simulink model "simulink_model"  (R2024a)
settings: Solver=VariableStepAuto  StartTime=0.0  StopTime=1  RelTol=1e-3
values from neighbouring files (symbols this model uses):
  control = set_control_gain(Kt_history(pid_count), input, control)    [Kd_tuner.m]    (also in Kd_tuner_newton.m = set_control_gain(Kt_history(pid_count)+delta_x, input, contr; target_tuner.m = set_control_gain(Kp_init, input, control))
undefined symbols (not defined in the file or in its folder): DiscIntNeverNeededParam, input, model
libraries: simulink x5, slpidlib x2
settings Model: PacingRate=0.010000  Creator=dionl  LastModifiedBy=dionl

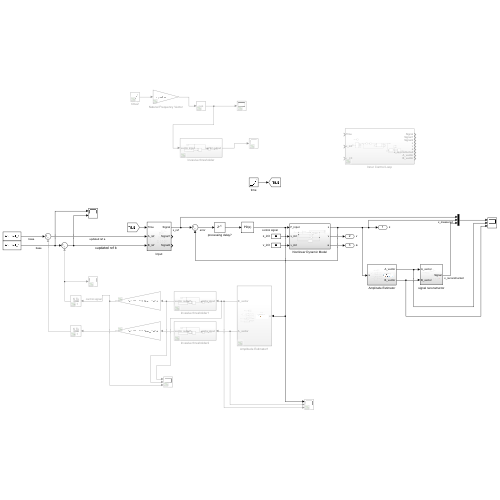
[thumbnail: Simulink's stored preview of the top-level diagram]
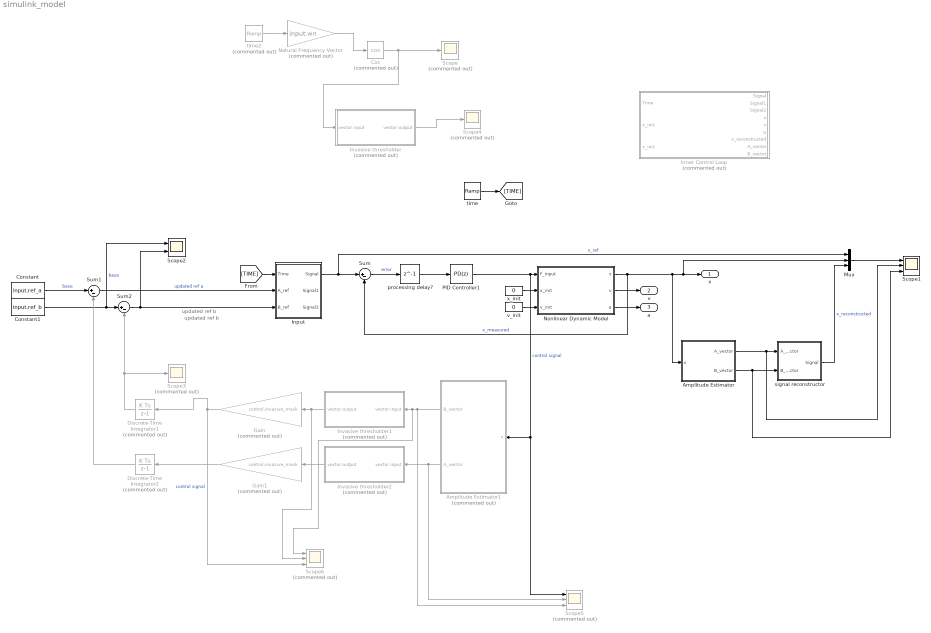
== system simulink_model ==
  note: updated ref b
  note: updated ref b
  Amplitude Estimator : Subsystem
  Amplitude Estimator1 : Subsystem  Commented=on
  Constant : Constant  Value=input.ref_a
  Constant1 : Constant  Value=input.ref_b
  Cos : Trigonometry  Commented=on  Operator=cos
  Discrete-Time Integrator1 : DiscreteIntegrator  Commented=on  SampleTime=input.T0*10  ICPrevOutput=DiscIntNeverNeededParam  ICPrevScaledInput=DiscIntNeverNeededParam
  Discrete-Time Integrator2 : DiscreteIntegrator  Commented=on  SampleTime=input.T0*10  ICPrevOutput=DiscIntNeverNeededParam  ICPrevScaledInput=DiscIntNeverNeededParam
  Gain : Gain  Commented=on  Gain=control.invasive_mask
  Gain1 : Gain  Commented=on  Gain=control.invasive_mask
  Inner Control Loop : Subsystem  Commented=on
  Input : Subsystem
  Invasive thresholder : Subsystem  Commented=on
  Invasive thresholder1 : Subsystem  Commented=on
  Invasive thresholder2 : Subsystem  Commented=on
  Mux : Mux  Inputs=3
  Natural Frequency Vector : Gain  Commented=on  Gain=input.wn
  Nonlinear Dynamic Model : Subsystem
  PID Controller1 : slpidlib/PID Controller  Controller=PD  Form=Parallel  TimeDomain=Discrete-time  UseExternalTs=off  SampleTime=control.Ts  IntegratorMethod=Forward Euler  FilterMethod=Forward Euler  ControllerParametersSource=internal  P=121287.822623306  I=152261.0112316  UseKiTs=off  D=51.5167470875525  UseExternalDerivativeSource=off  N=10629.0819573612  UseFilter=on  TunerSelectOption=Transfer Function Based (PID Tuner App)  InitialConditionSource=internal  InitialConditionForIntegrator=0  InitialConditionForFilter=0  DifferentiatorICPrevScaledInput=0  ExternalReset=none  TrackingMode=off  Kt=1  LimitOutput=off  SatLimitsSource=internal  UpperSaturationLimit=inf  LowerSaturationLimit=-inf  LinearizeAsGain=on  AntiWindupMode=none  Kb=1  LimitIntegrator=off  UpperIntegratorSaturationLimit=inf  LowerIntegratorSaturationLimit=-inf  POutMin=[]  POutMax=[]  IOutMin=[]  IOutMax=[]  DOutMin=[]  DOutMax=[]  NOutMin=[]  NOutMax=[]  SumOutMin=[]  SumOutMax=[]  SaturationOutMin=[]  SaturationOutMax=[]  PParamMin=[]  PParamMax=[]  IParamMin=[]  IParamMax=[]  DParamMin=[]  DParamMax=[]  NParamMin=[]  NParamMax=[]  KbParamMin=[]  KbParamMax=[]  KtParamMin=[]  KtParamMax=[]  KbOutMin=[]  KbOutMax=[]  KtOutMin=[]  KtOutMax=[]  IntegratorOutMin=[]  IntegratorOutMax=[]  FilterOutMin=[]  FilterOutMax=[]  SumI1OutMin=[]  SumI1OutMax=[]  SumI2OutMin=[]  SumI2OutMax=[]  SumI3OutMin=[]  SumI3OutMax=[]  SumI4OutMin=[]  SumI4OutMax=[]  SumDOutMin=[]  SumDOutMax=[]  DifferentiatorOutMin=[]  DifferentiatorOutMax=[]  FilterDiffOutCoefMin=[]  FilterDiffOutCoefMax=[]  ReciprocalOutMin=[]  ReciprocalOutMax=[]  SumDenOutMin=[]  SumDenOutMax=[]  SumNumOutMin=[]  SumNumOutMax=[]  DivideOutMin=[]  DivideOutMax=[]  UdiffTsProdOutMin=[]  UdiffTsProdOutMax=[]  NTsProdOutMin=[]  NTsProdOutMax=[]  UintegralTsProdOutMin=[]  UintegralTsProdOutMax=[]  UngainTsProdOutMin=[]  UngainTsProdOutMax=[]  ClampingZeroOutDataTypeStr=Inherit: Inherit via back propagation  ClampingZeroOutMin=[]  ClampingZeroOutMax=[]  FilterDenConstantOutDataTypeStr=Inherit: Inherit via back propagation  FilterDenConstantOutMin=[]  FilterDenConstantOutMax=[]  PCopyOutDataTypeStr=Inherit: Inherit via back propagation  PCopyOutMin=[]  PCopyOutMax=[]  NCopyOutDataTypeStr=Inherit: Inherit via back propagation  NCopyOutMin=[]  NCopyOutMax=[]  IntegratorContinuousStateAttributes=''  IntegratorStateMustResolveToSignalObject=off  IntegratorRTWStateStorageClass=Auto  FilterContinuousStateAttributes=''  FilterStateMustResolveToSignalObject=off  FilterRTWStateStorageClass=Auto  ParallelPVariant=InternalParameters  IdealPVariant=Disabled  IVariant=InternalParameters  DVariant=InternalParameters  IntegratorVariant=Continuous  SatVariant=Disabled  AWVariant=Passthrough  PCopyVariant=Disabled  TRVariant=Disabled  FdbkBlocksVariant=Forward  IdealPFdbkVariant=Disabled  SatFdbkVariant=Disabled  DerivativeFilterVariant=ContFilter  NVariant=InternalParameters  NCopyVariant=Disabled  FilterICVariant=InternalICsFilter  IntegratorICVariant=InternalICs  ExternalResetVariant=Disabled  TRSumVariant=Passthrough  SumFdbkVariant=Disabled  SumVariant=Sum_PID  TsampFilterVariant=InternalTs  TsampNgainVariant=Passthrough  TsampIntegralVariant=Passthrough  ExternalSaturationOutDataTypeStr=Inherit: Same as second input  DerivativeSourceVariant=ErrorSignal
  Scope : Scope  Commented=on
  Scope1 : Scope  NumInputPorts=3
  Scope2 : Scope  NumInputPorts=2
  Scope3 : Scope  Commented=on
  Scope4 : Scope  Commented=on
  Scope5 : Scope  Commented=on  NumInputPorts=3
  Scope6 : Scope  Commented=on  NumInputPorts=3
  Sum : Sum  Inputs=|+-
  Sum1 : Sum  Inputs=|+-
  Sum2 : Sum  Inputs=|+-
  processing delay? : Delay  DelayLength=1  SampleTime=control.Ts
  signal reconstructor : Subsystem
  time : simulink/Sources/Ramp  slope=1  start=0  InitialOutput=0
  time2 : simulink/Sources/Ramp  Commented=on  slope=1  start=0  InitialOutput=0
  v_init : Constant  Value=0
  x_init : Constant  Value=0
  x : Outport
  v : Outport  Port=2
  a : Outport  Port=3
  wires:
  Nonlinear Dynamic Model/3(a) -> a/1
  x_init/1 -> Nonlinear Dynamic Model/2(x_init)
  v_init/1 -> Nonlinear Dynamic Model/3(v_init)
  Nonlinear Dynamic Model/1(x) -> Sum/2, Amplitude Estimator/1(x), Mux/2, x/1  "x_measured"
  time/1 -> [TIME]
  Input/1(Signal) -> Mux/1, Sum/1  "x_ref"
  Nonlinear Dynamic Model/2(v) -> v/1
  Amplitude Estimator/1(A_vector) -> signal reconstructor/1(A_vector), Scope1/2
  Amplitude Estimator/2(B_vector) -> Scope1/3, signal reconstructor/2(B_vector)
  signal reconstructor/1(Signal) -> Mux/3  "x_reconstructed"
  Mux/1 -> Scope1/1
  Sum/1 -> processing delay?/1  "error"
  PID Controller1/1 -> Scope5/1, Amplitude Estimator1/1(x), Nonlinear Dynamic Model/1(F_input)  "control signal"
  processing delay?/1 -> PID Controller1/1
  [TIME] -> Input/1(Time)
  Constant/1 -> Sum1/1  "base"
  Sum1/1 -> Input/2(A_ref)  "updated ref a"
  Sum2/1 -> Scope2/2, Input/3(B_ref)
  Constant1/1 -> Scope2/1, Sum2/1  "base"
  Discrete-Time Integrator1/1 -> Scope3/1, Sum2/2
  Gain1/1 -> Discrete-Time Integrator2/1
  Discrete-Time Integrator2/1 -> Sum1/2
  Natural Frequency Vector/1 -> Cos/1
  time2/1 -> Natural Frequency Vector/1
  Cos/1 -> Invasive thresholder/1(vector input), Scope/1
  Invasive thresholder/1(vector output) -> Scope4/1
  Invasive thresholder1/1(vector output) -> Scope6/2, Gain/1
  Invasive thresholder2/1(vector output) -> Gain1/1
  Amplitude Estimator1/2(A_vector) -> Invasive thresholder2/1(vector input), Scope5/2
  Amplitude Estimator1/1(B_vector) -> Scope5/3, Scope6/1, Invasive thresholder1/1(vector input)
  Gain/1 -> Discrete-Time Integrator1/1, Scope6/3  "control signal"

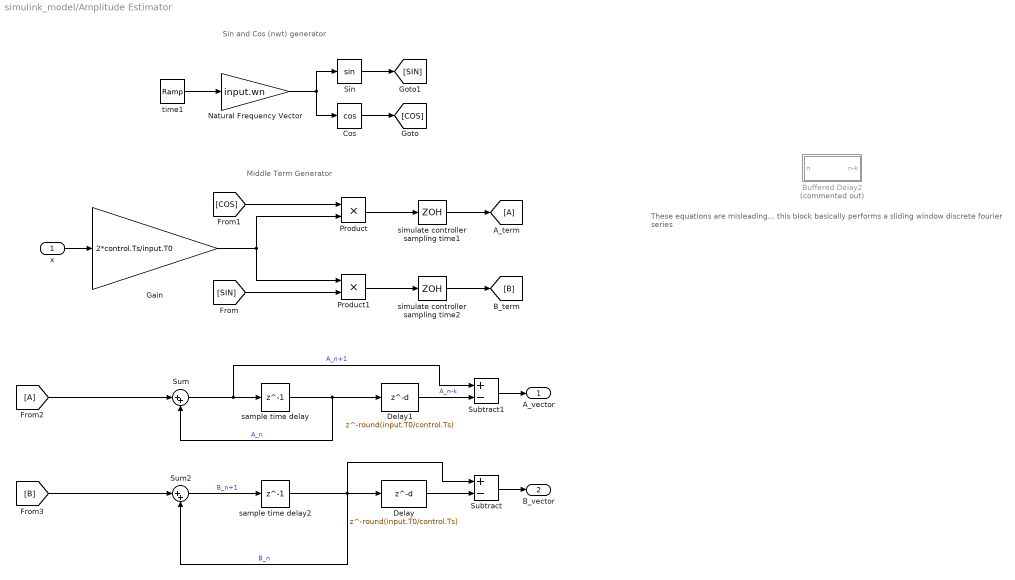
== system simulink_model/Amplitude Estimator ==
  note: These equations are misleading...
      | this block basically performs a sliding window discrete fourier series
  note: Sin and Cos (nwt) generator
  note: Middle Term Generator
  x : Inport
  A_term : Goto
  Buffered Delay2 : Subsystem  Commented=on
  Cos : Trigonometry  Operator=cos
  Delay : Delay  DelayLength=round(input.T0/control.Ts)  SampleTime=control.Ts
  Delay1 : Delay  DelayLength=round(input.T0/control.Ts)  SampleTime=control.Ts
  From2 : From
  Gain : Gain  Gain=2*control.Ts/input.T0
  Natural Frequency Vector : Gain  Gain=input.wn
  Product : Product
  Product1 : Product
  Sin : Trigonometry
  Subtract : Sum  Inputs=+-
  Subtract1 : Sum  Inputs=+-
  Sum : Sum  Inputs=|++
  Sum2 : Sum  Inputs=|++
  sample time delay : Delay  DelayLength=1  SampleTime=control.Ts
  sample time delay2 : Delay  DelayLength=1  SampleTime=control.Ts
  simulate controller sampling time1 : ZeroOrderHold  SampleTime=control.Ts
  simulate controller sampling time2 : ZeroOrderHold  SampleTime=control.Ts
  time1 : simulink/Sources/Ramp  slope=1  start=0  InitialOutput=0
  A_vector : Outport
  B_vector : Outport  Port=2
  wires:
  x/1 -> Gain/1
  time1/1 -> Natural Frequency Vector/1
  Natural Frequency Vector/1 -> Cos/1, Sin/1
  Sin/1 -> [SIN]
  Cos/1 -> [COS]
  [COS] -> Product/1
  Gain/1 -> Product1/1, Product/2
  [SIN] -> Product1/2
  Product/1 -> simulate controller sampling time1/1
  Product1/1 -> simulate controller sampling time2/1
  Sum/1 -> Subtract1/1, sample time delay/1  "A_n+1"
  sample time delay/1 -> Delay1/1, Sum/2  "A_n"
  Delay1/1 -> Subtract1/2  "A_n-k"
  From2/1 -> Sum/1
  [B] -> Sum2/1
  Delay/1 -> Subtract/2
  sample time delay2/1 -> Delay/1, Subtract/1, Sum2/2  "B_n"
  Sum2/1 -> sample time delay2/1  "B_n+1"
  simulate controller sampling time1/1 -> A_term/1
  simulate controller sampling time2/1 -> [B]
  Subtract/1 -> B_vector/1
  Subtract1/1 -> A_vector/1

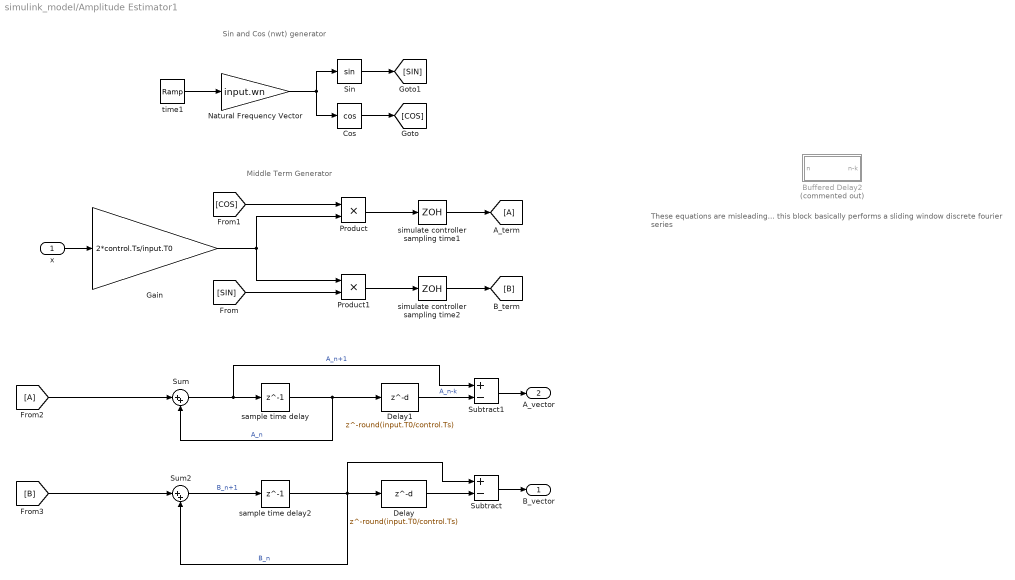
== system simulink_model/Amplitude Estimator1 ==
  note: Middle Term Generator
  note: Sin and Cos (nwt) generator
  note: These equations are misleading...
      | this block basically performs a sliding window discrete fourier series
  x : Inport
  A_term : Goto
  Buffered Delay2 : Subsystem  Commented=on
  Cos : Trigonometry  Operator=cos
  Delay : Delay  DelayLength=round(input.T0/control.Ts)  SampleTime=control.Ts
  Delay1 : Delay  DelayLength=round(input.T0/control.Ts)  SampleTime=control.Ts
  From2 : From
  Gain : Gain  Gain=2*control.Ts/input.T0
  Natural Frequency Vector : Gain  Gain=input.wn
  Product : Product
  Product1 : Product
  Sin : Trigonometry
  Subtract : Sum  Inputs=+-
  Subtract1 : Sum  Inputs=+-
  Sum : Sum  Inputs=|++
  Sum2 : Sum  Inputs=|++
  sample time delay : Delay  DelayLength=1  SampleTime=control.Ts
  sample time delay2 : Delay  DelayLength=1  SampleTime=control.Ts
  simulate controller sampling time1 : ZeroOrderHold  SampleTime=control.Ts
  simulate controller sampling time2 : ZeroOrderHold  SampleTime=control.Ts
  time1 : simulink/Sources/Ramp  slope=1  start=0  InitialOutput=0
  B_vector : Outport
  A_vector : Outport  Port=2
  wires:
  Subtract1/1 -> A_vector/1
  Subtract/1 -> B_vector/1
  simulate controller sampling time2/1 -> [B]
  simulate controller sampling time1/1 -> A_term/1
  Sum2/1 -> sample time delay2/1  "B_n+1"
  sample time delay2/1 -> Sum2/2, Subtract/1, Delay/1  "B_n"
  Delay/1 -> Subtract/2
  [B] -> Sum2/1
  From2/1 -> Sum/1
  Delay1/1 -> Subtract1/2  "A_n-k"
  sample time delay/1 -> Sum/2, Delay1/1  "A_n"
  Sum/1 -> sample time delay/1, Subtract1/1  "A_n+1"
  Product1/1 -> simulate controller sampling time2/1
  Product/1 -> simulate controller sampling time1/1
  [SIN] -> Product1/2
  Gain/1 -> Product/2, Product1/1
  [COS] -> Product/1
  Cos/1 -> [COS]
  Sin/1 -> [SIN]
  Natural Frequency Vector/1 -> Sin/1, Cos/1
  time1/1 -> Natural Frequency Vector/1
  x/1 -> Gain/1

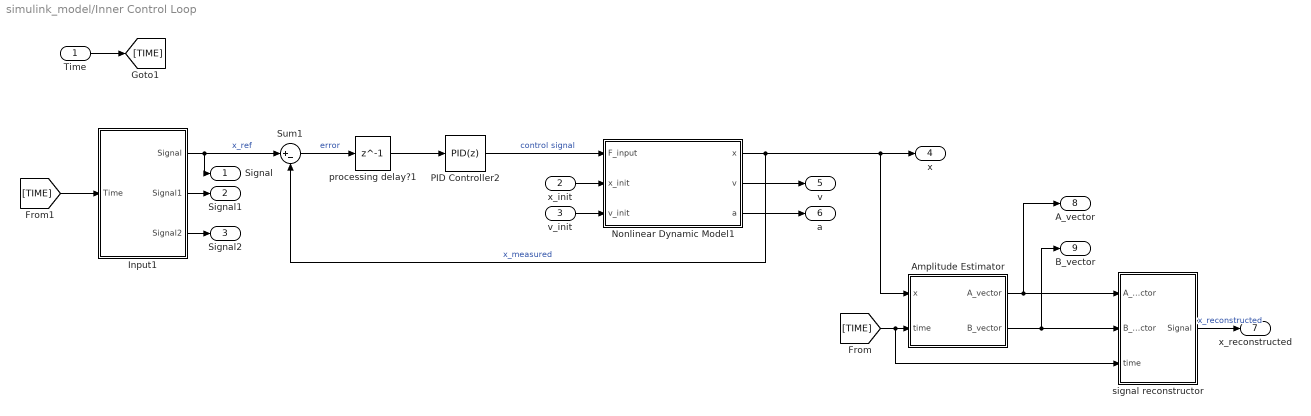
== system simulink_model/Inner Control Loop ==
  Time : Inport
  x_init : Inport  Port=2
  v_init : Inport  Port=3
  Amplitude Estimator : Subsystem
  Input1 : Subsystem
  Nonlinear Dynamic Model1 : Subsystem
  PID Controller2 : slpidlib/PID Controller  Controller=PID  Form=Parallel  TimeDomain=Discrete-time  UseExternalTs=off  SampleTime=control.Ts  IntegratorMethod=Forward Euler  FilterMethod=Forward Euler  ControllerParametersSource=internal  P=539.321576217819  I=451.426183923391  UseKiTs=off  D=143.042872882207  UseExternalDerivativeSource=off  N=1782.65180383031  UseFilter=on  TunerSelectOption=Transfer Function Based (PID Tuner App)  InitialConditionSource=internal  InitialConditionForIntegrator=0  InitialConditionForFilter=0  DifferentiatorICPrevScaledInput=0  ExternalReset=none  TrackingMode=off  Kt=1  LimitOutput=off  SatLimitsSource=internal  UpperSaturationLimit=inf  LowerSaturationLimit=-inf  LinearizeAsGain=on  AntiWindupMode=none  Kb=1  LimitIntegrator=off  UpperIntegratorSaturationLimit=inf  LowerIntegratorSaturationLimit=-inf  POutMin=[]  POutMax=[]  IOutMin=[]  IOutMax=[]  DOutMin=[]  DOutMax=[]  NOutMin=[]  NOutMax=[]  SumOutMin=[]  SumOutMax=[]  SaturationOutMin=[]  SaturationOutMax=[]  PParamMin=[]  PParamMax=[]  IParamMin=[]  IParamMax=[]  DParamMin=[]  DParamMax=[]  NParamMin=[]  NParamMax=[]  KbParamMin=[]  KbParamMax=[]  KtParamMin=[]  KtParamMax=[]  KbOutMin=[]  KbOutMax=[]  KtOutMin=[]  KtOutMax=[]  IntegratorOutMin=[]  IntegratorOutMax=[]  FilterOutMin=[]  FilterOutMax=[]  SumI1OutMin=[]  SumI1OutMax=[]  SumI2OutMin=[]  SumI2OutMax=[]  SumI3OutMin=[]  SumI3OutMax=[]  SumI4OutMin=[]  SumI4OutMax=[]  SumDOutMin=[]  SumDOutMax=[]  DifferentiatorOutMin=[]  DifferentiatorOutMax=[]  FilterDiffOutCoefMin=[]  FilterDiffOutCoefMax=[]  ReciprocalOutMin=[]  ReciprocalOutMax=[]  SumDenOutMin=[]  SumDenOutMax=[]  SumNumOutMin=[]  SumNumOutMax=[]  DivideOutMin=[]  DivideOutMax=[]  UdiffTsProdOutMin=[]  UdiffTsProdOutMax=[]  NTsProdOutMin=[]  NTsProdOutMax=[]  UintegralTsProdOutMin=[]  UintegralTsProdOutMax=[]  UngainTsProdOutMin=[]  UngainTsProdOutMax=[]  ClampingZeroOutDataTypeStr=Inherit: Inherit via back propagation  ClampingZeroOutMin=[]  ClampingZeroOutMax=[]  FilterDenConstantOutDataTypeStr=Inherit: Inherit via back propagation  FilterDenConstantOutMin=[]  FilterDenConstantOutMax=[]  PCopyOutDataTypeStr=Inherit: Inherit via back propagation  PCopyOutMin=[]  PCopyOutMax=[]  NCopyOutDataTypeStr=Inherit: Inherit via back propagation  NCopyOutMin=[]  NCopyOutMax=[]  IntegratorContinuousStateAttributes=''  IntegratorStateMustResolveToSignalObject=off  IntegratorRTWStateStorageClass=Auto  FilterContinuousStateAttributes=''  FilterStateMustResolveToSignalObject=off  FilterRTWStateStorageClass=Auto  ParallelPVariant=InternalParameters  IdealPVariant=Disabled  IVariant=InternalParameters  DVariant=InternalParameters  IntegratorVariant=Continuous  SatVariant=Disabled  AWVariant=Passthrough  PCopyVariant=Disabled  TRVariant=Disabled  FdbkBlocksVariant=Forward  IdealPFdbkVariant=Disabled  SatFdbkVariant=Disabled  DerivativeFilterVariant=ContFilter  NVariant=InternalParameters  NCopyVariant=Disabled  FilterICVariant=InternalICsFilter  IntegratorICVariant=InternalICs  ExternalResetVariant=Disabled  TRSumVariant=Passthrough  SumFdbkVariant=Disabled  SumVariant=Sum_PID  TsampFilterVariant=InternalTs  TsampNgainVariant=Passthrough  TsampIntegralVariant=Passthrough  ExternalSaturationOutDataTypeStr=Inherit: Same as second input  DerivativeSourceVariant=ErrorSignal
  Sum1 : Sum  Inputs=|+-
  processing delay?1 : Delay  DelayLength=1  SampleTime=control.Ts
  signal reconstructor : Subsystem
  Signal : Outport
  Signal1 : Outport  Port=2
  Signal2 : Outport  Port=3
  x : Outport  Port=4
  v : Outport  Port=5
  a : Outport  Port=6
  x_reconstructed : Outport  Port=7
  A_vector : Outport  Port=8
  B_vector : Outport  Port=9
  wires:
  Sum1/1 -> processing delay?1/1  "error"
  Time/1 -> [TIME]
  Nonlinear Dynamic Model1/1(x) -> Sum1/2, Amplitude Estimator/1(x), x/1  "x_measured"
  PID Controller2/1 -> Nonlinear Dynamic Model1/1(F_input)  "control signal"
  processing delay?1/1 -> PID Controller2/1
  Input1/2(Signal1) -> Signal1/1
  x_init/1 -> Nonlinear Dynamic Model1/2(x_init)
  Amplitude Estimator/2(B_vector) -> signal reconstructor/2(B_vector), B_vector/1
  Input1/3(Signal2) -> Signal2/1
  Amplitude Estimator/1(A_vector) -> A_vector/1, signal reconstructor/1(A_vector)
  Input1/1(Signal) -> Signal/1, Sum1/1  "x_ref"
  v_init/1 -> Nonlinear Dynamic Model1/3(v_init)
  Nonlinear Dynamic Model1/2(v) -> v/1
  Nonlinear Dynamic Model1/3(a) -> a/1
  [TIME] -> Input1/1(Time)
  [TIME] -> signal reconstructor/3(time), Amplitude Estimator/2(time)
  signal reconstructor/1(Signal) -> x_reconstructed/1  "x_reconstructed"

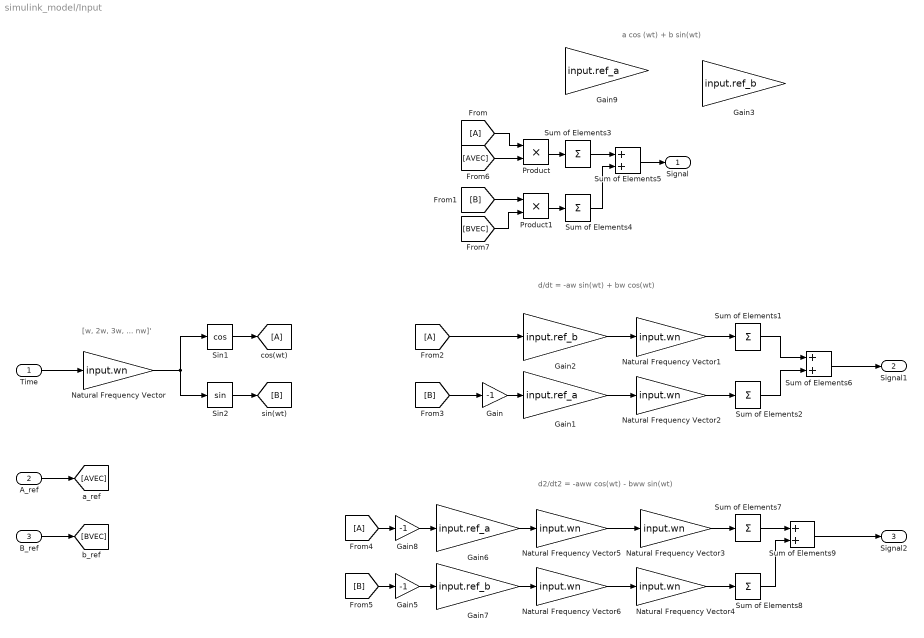
== system simulink_model/Input ==
  note: a cos (wt) + b sin(wt)
  note: d2/dt2 = -aww cos(wt) - bww sin(wt)
  note: d/dt = -aw sin(wt) + bw cos(wt)
  note: [w, 2w, 3w, ... nw]'
  Time : Inport
  A_ref : Inport  Port=2
  B_ref : Inport  Port=3
  From : From
  From2 : From
  From4 : From
  Gain : Gain  Gain=-1
  Gain1 : Gain  Gain=input.ref_a
  Gain2 : Gain  Gain=input.ref_b
  Gain3 : Gain  Gain=input.ref_b
  Gain5 : Gain  Gain=-1
  Gain6 : Gain  Gain=input.ref_a
  Gain7 : Gain  Gain=input.ref_b
  Gain8 : Gain  Gain=-1
  Gain9 : Gain  Gain=input.ref_a
  Natural Frequency Vector{,1..6} (7 alike) : Gain  Gain=input.wn
  Product : Product
  Product1 : Product
  Sin1 : Trigonometry  Operator=cos
  Sin2 : Trigonometry
  Sum of Elements{1..4,7..8} (6 alike) : Sum  Inputs=+
  Sum of Elements5 : Sum
  Sum of Elements6 : Sum
  Sum of Elements9 : Sum
  cos(wt) : Goto
  Signal : Outport
  Signal1 : Outport  Port=2
  Signal2 : Outport  Port=3
  wires:
  Time/1 -> Natural Frequency Vector/1
  Sin1/1 -> cos(wt)/1
  Sin2/1 -> [B]
  Natural Frequency Vector/1 -> Sin1/1, Sin2/1
  [B] -> Product1/1
  Sum of Elements3/1 -> Sum of Elements5/1
  Sum of Elements4/1 -> Sum of Elements5/2
  Sum of Elements5/1 -> Signal/1
  From/1 -> Product/1
  Product/1 -> Sum of Elements3/1
  Product1/1 -> Sum of Elements4/1
  [B] -> Gain/1
  Gain/1 -> Gain1/1
  Gain1/1 -> Natural Frequency Vector2/1
  Gain2/1 -> Natural Frequency Vector1/1
  From2/1 -> Gain2/1
  Natural Frequency Vector1/1 -> Sum of Elements1/1
  Natural Frequency Vector2/1 -> Sum of Elements2/1
  Sum of Elements1/1 -> Sum of Elements6/1
  Sum of Elements2/1 -> Sum of Elements6/2
  Sum of Elements9/1 -> Signal2/1
  Sum of Elements8/1 -> Sum of Elements9/2
  Sum of Elements7/1 -> Sum of Elements9/1
  Natural Frequency Vector4/1 -> Sum of Elements8/1
  Natural Frequency Vector3/1 -> Sum of Elements7/1
  From4/1 -> Gain8/1
  Natural Frequency Vector5/1 -> Natural Frequency Vector3/1
  Natural Frequency Vector6/1 -> Natural Frequency Vector4/1
  [B] -> Gain5/1
  Gain8/1 -> Gain6/1
  Gain6/1 -> Natural Frequency Vector5/1
  Gain5/1 -> Gain7/1
  Gain7/1 -> Natural Frequency Vector6/1
  Sum of Elements6/1 -> Signal1/1
  A_ref/1 -> [AVEC]
  B_ref/1 -> [BVEC]
  [AVEC] -> Product/2
  [BVEC] -> Product1/2

== system simulink_model/Invasive thresholder ==
  vector input : Inport
  Constant3 : Constant  Value=control.invasive_threshold
  GreaterThan : RelationalOperator  Operator=>  OutDataTypeStr=boolean  RndMeth=Simplest  InputSameDT=off
  Product : Product
  vector output : Outport
  wires:
  GreaterThan/1 -> Product/2
  vector input/1 -> Product/1, GreaterThan/1
  Product/1 -> vector output/1
  Constant3/1 -> GreaterThan/2

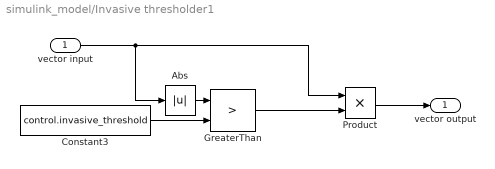
== system simulink_model/Invasive thresholder1 ==
  vector input : Inport
  Abs : Abs  SaturateOnIntegerOverflow=off
  Constant3 : Constant  Value=control.invasive_threshold
  GreaterThan : RelationalOperator  Operator=>  OutDataTypeStr=boolean  RndMeth=Simplest  InputSameDT=off
  Product : Product
  vector output : Outport
  wires:
  GreaterThan/1 -> Product/2
  vector input/1 -> Abs/1, Product/1
  Product/1 -> vector output/1
  Constant3/1 -> GreaterThan/2
  Abs/1 -> GreaterThan/1

== system simulink_model/Invasive thresholder2 ==
  vector input : Inport
  Abs : Abs  SaturateOnIntegerOverflow=off
  Constant3 : Constant  Value=control.invasive_threshold
  GreaterThan : RelationalOperator  Operator=>  OutDataTypeStr=boolean  RndMeth=Simplest  InputSameDT=off
  Product : Product
  vector output : Outport
  wires:
  Abs/1 -> GreaterThan/1
  Constant3/1 -> GreaterThan/2
  Product/1 -> vector output/1
  vector input/1 -> Product/1, Abs/1
  GreaterThan/1 -> Product/2

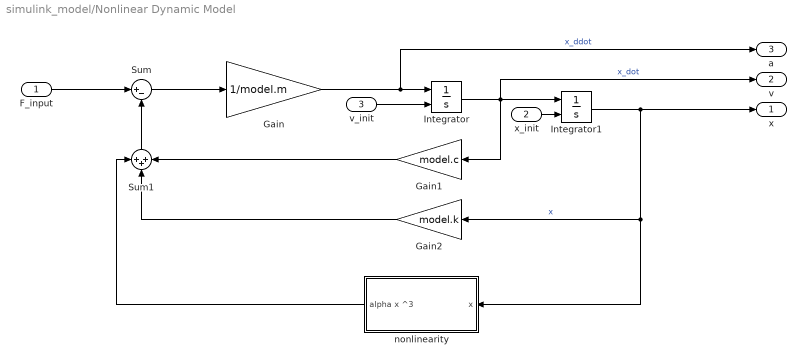
== system simulink_model/Nonlinear Dynamic Model ==
  F_input : Inport
  x_init : Inport  Port=2
  v_init : Inport  Port=3
  Gain : Gain  Gain=1/model.m
  Gain1 : Gain  Gain=model.c
  Gain2 : Gain  Gain=model.k
  Integrator : Integrator  InitialConditionSource=external
  Integrator1 : Integrator  InitialConditionSource=external
  Sum : Sum  Inputs=|+-
  Sum1 : Sum  Inputs=+++
  nonlinearity : Subsystem
  x : Outport
  v : Outport  Port=2
  a : Outport  Port=3
  wires:
  Gain/1 -> a/1, Integrator/1  "x_ddot"
  Sum1/1 -> Sum/2
  Gain2/1 -> Sum1/2
  x_init/1 -> Integrator1/2
  F_input/1 -> Sum/1
  nonlinearity/1(alpha x ^3) -> Sum1/1
  Sum/1 -> Gain/1
  Integrator1/1 -> x/1, nonlinearity/1(x), Gain2/1  "x"
  Integrator/1 -> v/1, Integrator1/1, Gain1/1  "x_dot"
  Gain1/1 -> Sum1/3
  v_init/1 -> Integrator/2

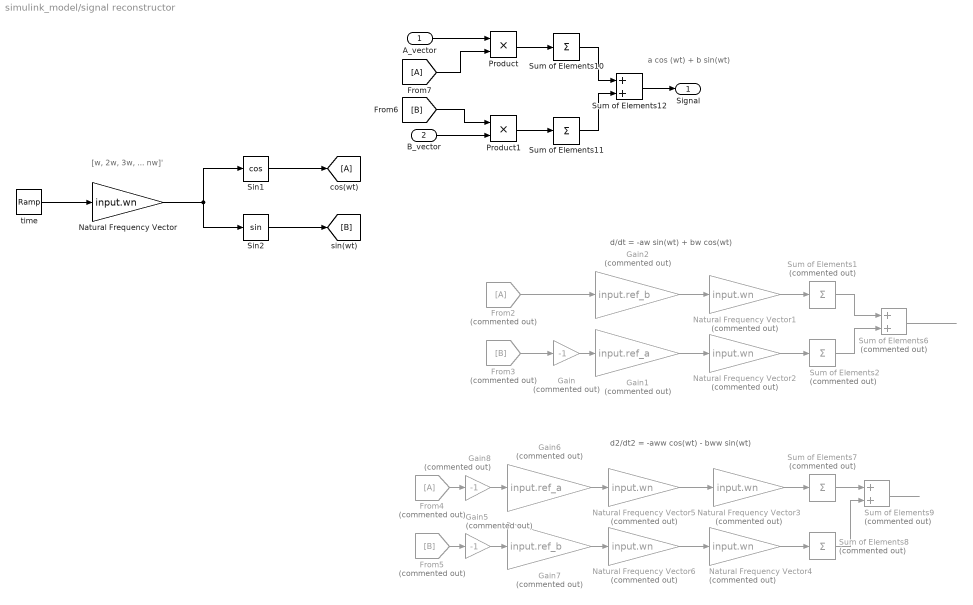
== system simulink_model/signal reconstructor ==
  note: [w, 2w, 3w, ... nw]'
  note: d/dt = -aw sin(wt) + bw cos(wt)
  note: d2/dt2 = -aww cos(wt) - bww sin(wt)
  note: a cos (wt) + b sin(wt)
  A_vector : Inport
  B_vector : Inport  Port=2
  From2 : From  Commented=on
  From3 : From  Commented=on  GotoTag=B
  From4 : From  Commented=on
  From5 : From  Commented=on  GotoTag=B
  From7 : From
  Gain : Gain  Commented=on  Gain=-1
  Gain1 : Gain  Commented=on  Gain=input.ref_a
  Gain2 : Gain  Commented=on  Gain=input.ref_b
  Gain5 : Gain  Commented=on  Gain=-1
  Gain6 : Gain  Commented=on  Gain=input.ref_a
  Gain7 : Gain  Commented=on  Gain=input.ref_b
  Gain8 : Gain  Commented=on  Gain=-1
  Natural Frequency Vector : Gain  Gain=input.wn
  Natural Frequency Vector{1..6} (6 alike) : Gain  Commented=on  Gain=input.wn
  Product : Product
  Product1 : Product
  Sin1 : Trigonometry  Operator=cos
  Sin2 : Trigonometry
  Sum of Elements{1..2,7..8} (4 alike) : Sum  Commented=on  Inputs=+
  Sum of Elements10 : Sum  Inputs=+
  Sum of Elements11 : Sum  Inputs=+
  Sum of Elements12 : Sum
  Sum of Elements6 : Sum  Commented=on
  Sum of Elements9 : Sum  Commented=on
  cos(wt) : Goto
  time : simulink/Sources/Ramp  slope=1  start=0  InitialOutput=0
  Signal : Outport
  wires:
  Sum of Elements6/1 -> ?
  Gain7/1 -> Natural Frequency Vector6/1
  Gain5/1 -> Gain7/1
  Gain6/1 -> Natural Frequency Vector5/1
  Gain8/1 -> Gain6/1
  From5/1 -> Gain5/1
  Natural Frequency Vector6/1 -> Natural Frequency Vector4/1
  Natural Frequency Vector5/1 -> Natural Frequency Vector3/1
  From4/1 -> Gain8/1
  Natural Frequency Vector3/1 -> Sum of Elements7/1
  Natural Frequency Vector4/1 -> Sum of Elements8/1
  Sum of Elements7/1 -> Sum of Elements9/1
  Sum of Elements8/1 -> Sum of Elements9/2
  Sum of Elements9/1 -> ?
  Sum of Elements2/1 -> Sum of Elements6/2
  Sum of Elements1/1 -> Sum of Elements6/1
  Natural Frequency Vector2/1 -> Sum of Elements2/1
  Natural Frequency Vector1/1 -> Sum of Elements1/1
  From2/1 -> Gain2/1
  Gain2/1 -> Natural Frequency Vector1/1
  Gain1/1 -> Natural Frequency Vector2/1
  Gain/1 -> Gain1/1
  From3/1 -> Gain/1
  Natural Frequency Vector/1 -> Sin2/1, Sin1/1
  Sin2/1 -> [B]
  Sin1/1 -> cos(wt)/1
  A_vector/1 -> Product/1
  B_vector/1 -> Product1/2
  [B] -> Product1/1
  From7/1 -> Product/2
  Product1/1 -> Sum of Elements11/1
  Product/1 -> Sum of Elements10/1
  Sum of Elements10/1 -> Sum of Elements12/1
  Sum of Elements11/1 -> Sum of Elements12/2
  Sum of Elements12/1 -> Signal/1
  time/1 -> Natural Frequency Vector/1

== system simulink_model/Amplitude Estimator/Buffered Delay2 ==
  note: This block will take an input vector (signal) and output
      | the delayed signal according to a vector delay
  n : Inport
  Constant4 : Constant  Value=round(input.Tn./control.Ts)'
  MATLAB Function1 : MATLAB Function  TreatAsAtomicUnit=on
  n-k : Outport
  wires:
  Constant4/1 -> MATLAB Function1/2(delay_vec)
  n/1 -> MATLAB Function1/1(signal)
  MATLAB Function1/1(y) -> n-k/1  "A_n-k"

== system simulink_model/Amplitude Estimator1/Buffered Delay2 ==
  note: This block will take an input vector (signal) and output
      | the delayed signal according to a vector delay
  n : Inport
  Constant4 : Constant  Value=round(input.Tn./control.Ts)'
  MATLAB Function1 : MATLAB Function  TreatAsAtomicUnit=on
  n-k : Outport
  wires:
  MATLAB Function1/1(y) -> n-k/1  "A_n-k"
  n/1 -> MATLAB Function1/1(signal)
  Constant4/1 -> MATLAB Function1/2(delay_vec)

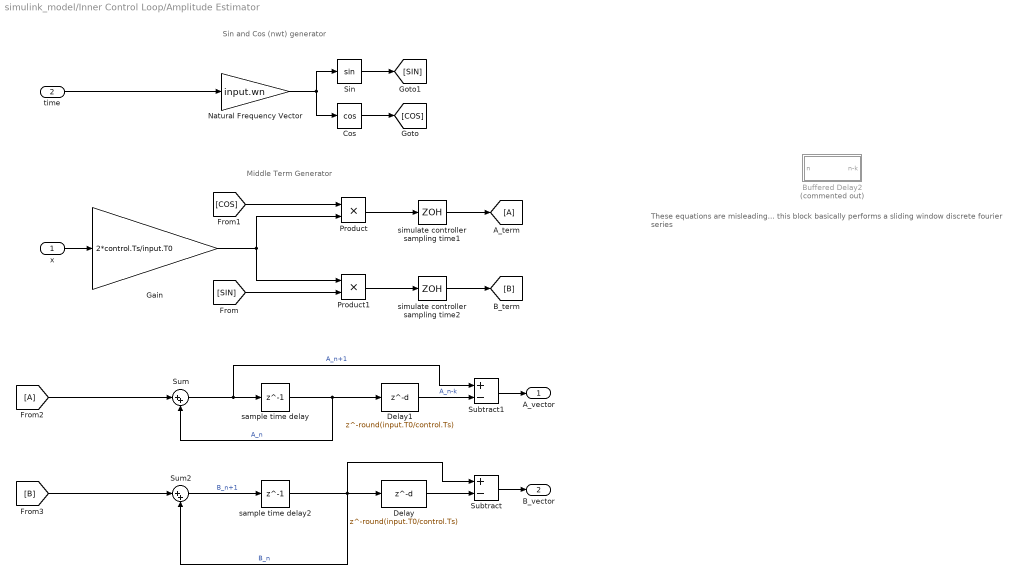
== system simulink_model/Inner Control Loop/Amplitude Estimator ==
  note: These equations are misleading...
      | this block basically performs a sliding window discrete fourier series
  note: Sin and Cos (nwt) generator
  note: Middle Term Generator
  x : Inport
  time : Inport  Port=2
  A_term : Goto
  Buffered Delay2 : Subsystem  Commented=on
  Cos : Trigonometry  Operator=cos
  Delay : Delay  DelayLength=round(input.T0/control.Ts)  SampleTime=control.Ts
  Delay1 : Delay  DelayLength=round(input.T0/control.Ts)  SampleTime=control.Ts
  From2 : From
  Gain : Gain  Gain=2*control.Ts/input.T0
  Natural Frequency Vector : Gain  Gain=input.wn
  Product : Product
  Product1 : Product
  Sin : Trigonometry
  Subtract : Sum  Inputs=+-
  Subtract1 : Sum  Inputs=+-
  Sum : Sum  Inputs=|++
  Sum2 : Sum  Inputs=|++
  sample time delay : Delay  DelayLength=1  SampleTime=control.Ts
  sample time delay2 : Delay  DelayLength=1  SampleTime=control.Ts
  simulate controller sampling time1 : ZeroOrderHold  SampleTime=control.Ts
  simulate controller sampling time2 : ZeroOrderHold  SampleTime=control.Ts
  A_vector : Outport
  B_vector : Outport  Port=2
  wires:
  x/1 -> Gain/1
  time/1 -> Natural Frequency Vector/1
  Natural Frequency Vector/1 -> Cos/1, Sin/1
  Sin/1 -> [SIN]
  Cos/1 -> [COS]
  [COS] -> Product/1
  Gain/1 -> Product1/1, Product/2
  [SIN] -> Product1/2
  Product/1 -> simulate controller sampling time1/1
  Product1/1 -> simulate controller sampling time2/1
  Sum/1 -> Subtract1/1, sample time delay/1  "A_n+1"
  sample time delay/1 -> Delay1/1, Sum/2  "A_n"
  Delay1/1 -> Subtract1/2  "A_n-k"
  From2/1 -> Sum/1
  [B] -> Sum2/1
  Delay/1 -> Subtract/2
  sample time delay2/1 -> Delay/1, Subtract/1, Sum2/2  "B_n"
  Sum2/1 -> sample time delay2/1  "B_n+1"
  simulate controller sampling time1/1 -> A_term/1
  simulate controller sampling time2/1 -> [B]
  Subtract/1 -> B_vector/1
  Subtract1/1 -> A_vector/1

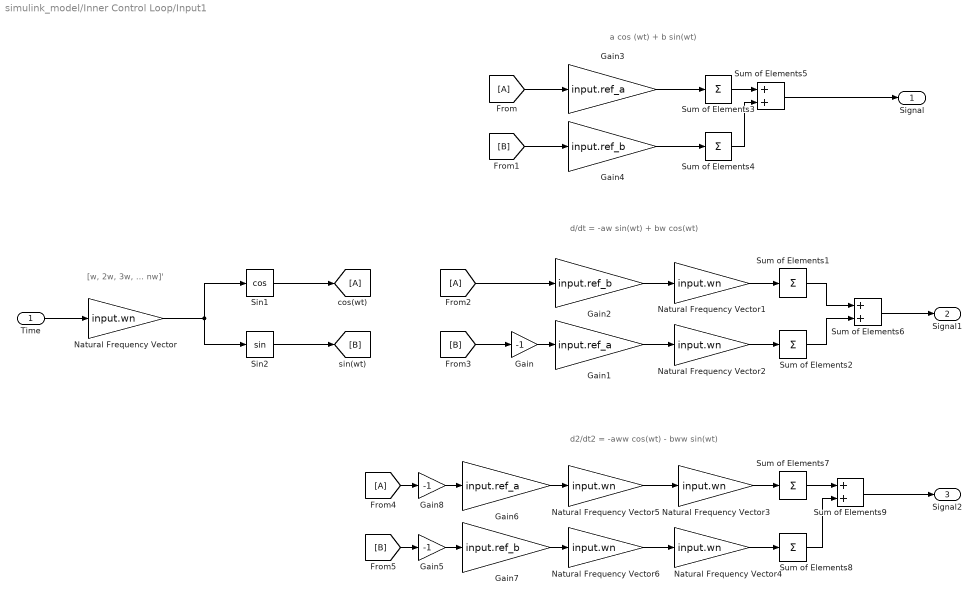
== system simulink_model/Inner Control Loop/Input1 ==
  note: a cos (wt) + b sin(wt)
  note: d2/dt2 = -aww cos(wt) - bww sin(wt)
  note: d/dt = -aw sin(wt) + bw cos(wt)
  note: [w, 2w, 3w, ... nw]'
  Time : Inport
  From : From
  From2 : From
  From4 : From
  Gain : Gain  Gain=-1
  Gain1 : Gain  Gain=input.ref_a
  Gain2 : Gain  Gain=input.ref_b
  Gain3 : Gain  Gain=input.ref_a
  Gain4 : Gain  Gain=input.ref_b
  Gain5 : Gain  Gain=-1
  Gain6 : Gain  Gain=input.ref_a
  Gain7 : Gain  Gain=input.ref_b
  Gain8 : Gain  Gain=-1
  Natural Frequency Vector{,1..6} (7 alike) : Gain  Gain=input.wn
  Sin1 : Trigonometry  Operator=cos
  Sin2 : Trigonometry
  Sum of Elements{1..4,7..8} (6 alike) : Sum  Inputs=+
  Sum of Elements5 : Sum
  Sum of Elements6 : Sum
  Sum of Elements9 : Sum
  cos(wt) : Goto
  Signal : Outport
  Signal1 : Outport  Port=2
  Signal2 : Outport  Port=3
  wires:
  Time/1 -> Natural Frequency Vector/1
  Sin1/1 -> cos(wt)/1
  Sin2/1 -> [B]
  Natural Frequency Vector/1 -> Sin1/1, Sin2/1
  [B] -> Gain4/1
  Sum of Elements3/1 -> Sum of Elements5/1
  Sum of Elements4/1 -> Sum of Elements5/2
  Sum of Elements5/1 -> Signal/1
  From/1 -> Gain3/1
  Gain3/1 -> Sum of Elements3/1
  Gain4/1 -> Sum of Elements4/1
  [B] -> Gain/1
  Gain/1 -> Gain1/1
  Gain1/1 -> Natural Frequency Vector2/1
  Gain2/1 -> Natural Frequency Vector1/1
  From2/1 -> Gain2/1
  Natural Frequency Vector1/1 -> Sum of Elements1/1
  Natural Frequency Vector2/1 -> Sum of Elements2/1
  Sum of Elements1/1 -> Sum of Elements6/1
  Sum of Elements2/1 -> Sum of Elements6/2
  Sum of Elements9/1 -> Signal2/1
  Sum of Elements8/1 -> Sum of Elements9/2
  Sum of Elements7/1 -> Sum of Elements9/1
  Natural Frequency Vector4/1 -> Sum of Elements8/1
  Natural Frequency Vector3/1 -> Sum of Elements7/1
  From4/1 -> Gain8/1
  Natural Frequency Vector5/1 -> Natural Frequency Vector3/1
  Natural Frequency Vector6/1 -> Natural Frequency Vector4/1
  [B] -> Gain5/1
  Gain8/1 -> Gain6/1
  Gain6/1 -> Natural Frequency Vector5/1
  Gain5/1 -> Gain7/1
  Gain7/1 -> Natural Frequency Vector6/1
  Sum of Elements6/1 -> Signal1/1

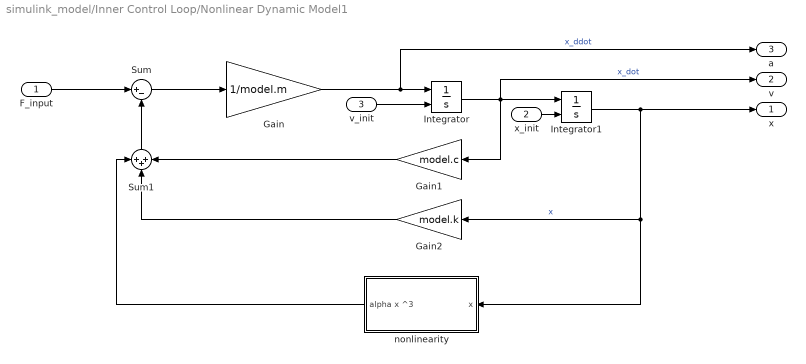
== system simulink_model/Inner Control Loop/Nonlinear Dynamic Model1 ==
  F_input : Inport
  x_init : Inport  Port=2
  v_init : Inport  Port=3
  Gain : Gain  Gain=1/model.m
  Gain1 : Gain  Gain=model.c
  Gain2 : Gain  Gain=model.k
  Integrator : Integrator  InitialConditionSource=external
  Integrator1 : Integrator  InitialConditionSource=external
  Sum : Sum  Inputs=|+-
  Sum1 : Sum  Inputs=+++
  nonlinearity : Subsystem
  x : Outport
  v : Outport  Port=2
  a : Outport  Port=3
  wires:
  Gain/1 -> a/1, Integrator/1  "x_ddot"
  Sum1/1 -> Sum/2
  Gain2/1 -> Sum1/2
  x_init/1 -> Integrator1/2
  F_input/1 -> Sum/1
  nonlinearity/1(alpha x ^3) -> Sum1/1
  Sum/1 -> Gain/1
  Integrator1/1 -> x/1, nonlinearity/1(x), Gain2/1  "x"
  Integrator/1 -> v/1, Integrator1/1, Gain1/1  "x_dot"
  Gain1/1 -> Sum1/3
  v_init/1 -> Integrator/2

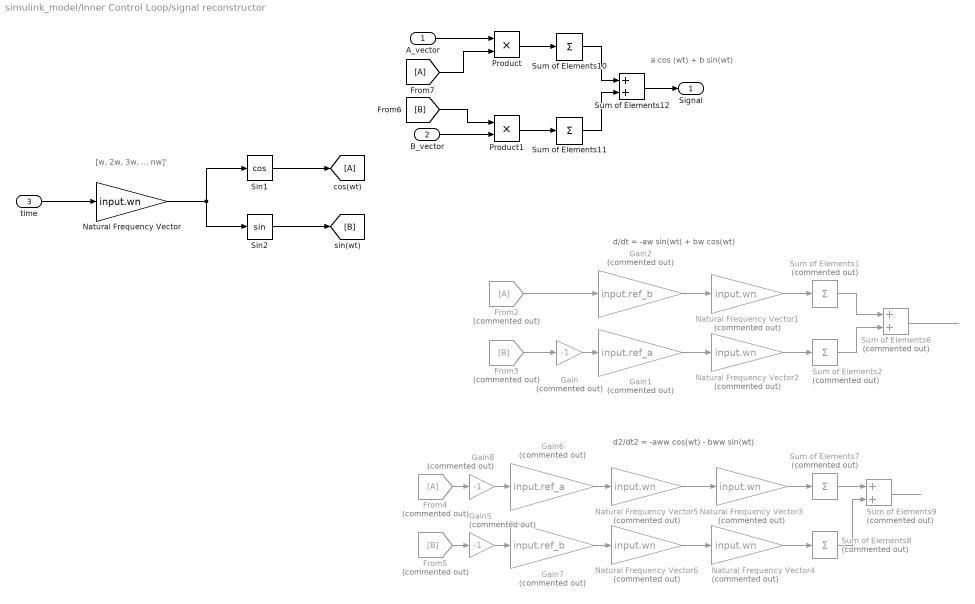
== system simulink_model/Inner Control Loop/signal reconstructor ==
  note: [w, 2w, 3w, ... nw]'
  note: d/dt = -aw sin(wt) + bw cos(wt)
  note: d2/dt2 = -aww cos(wt) - bww sin(wt)
  note: a cos (wt) + b sin(wt)
  A_vector : Inport
  B_vector : Inport  Port=2
  time : Inport  Port=3
  From2 : From  Commented=on
  From3 : From  Commented=on  GotoTag=B
  From4 : From  Commented=on
  From5 : From  Commented=on  GotoTag=B
  From7 : From
  Gain : Gain  Commented=on  Gain=-1
  Gain1 : Gain  Commented=on  Gain=input.ref_a
  Gain2 : Gain  Commented=on  Gain=input.ref_b
  Gain5 : Gain  Commented=on  Gain=-1
  Gain6 : Gain  Commented=on  Gain=input.ref_a
  Gain7 : Gain  Commented=on  Gain=input.ref_b
  Gain8 : Gain  Commented=on  Gain=-1
  Natural Frequency Vector : Gain  Gain=input.wn
  Natural Frequency Vector{1..6} (6 alike) : Gain  Commented=on  Gain=input.wn
  Product : Product
  Product1 : Product
  Sin1 : Trigonometry  Operator=cos
  Sin2 : Trigonometry
  Sum of Elements{1..2,7..8} (4 alike) : Sum  Commented=on  Inputs=+
  Sum of Elements10 : Sum  Inputs=+
  Sum of Elements11 : Sum  Inputs=+
  Sum of Elements12 : Sum
  Sum of Elements6 : Sum  Commented=on
  Sum of Elements9 : Sum  Commented=on
  cos(wt) : Goto
  Signal : Outport
  wires:
  Sum of Elements6/1 -> ?
  Gain7/1 -> Natural Frequency Vector6/1
  Gain5/1 -> Gain7/1
  Gain6/1 -> Natural Frequency Vector5/1
  Gain8/1 -> Gain6/1
  From5/1 -> Gain5/1
  Natural Frequency Vector6/1 -> Natural Frequency Vector4/1
  Natural Frequency Vector5/1 -> Natural Frequency Vector3/1
  From4/1 -> Gain8/1
  Natural Frequency Vector3/1 -> Sum of Elements7/1
  Natural Frequency Vector4/1 -> Sum of Elements8/1
  Sum of Elements7/1 -> Sum of Elements9/1
  Sum of Elements8/1 -> Sum of Elements9/2
  Sum of Elements9/1 -> ?
  Sum of Elements2/1 -> Sum of Elements6/2
  Sum of Elements1/1 -> Sum of Elements6/1
  Natural Frequency Vector2/1 -> Sum of Elements2/1
  Natural Frequency Vector1/1 -> Sum of Elements1/1
  From2/1 -> Gain2/1
  Gain2/1 -> Natural Frequency Vector1/1
  Gain1/1 -> Natural Frequency Vector2/1
  Gain/1 -> Gain1/1
  From3/1 -> Gain/1
  Natural Frequency Vector/1 -> Sin2/1, Sin1/1
  Sin2/1 -> [B]
  Sin1/1 -> cos(wt)/1
  A_vector/1 -> Product/1
  B_vector/1 -> Product1/2
  [B] -> Product1/1
  From7/1 -> Product/2
  Product1/1 -> Sum of Elements11/1
  Product/1 -> Sum of Elements10/1
  Sum of Elements10/1 -> Sum of Elements12/1
  Sum of Elements11/1 -> Sum of Elements12/2
  Sum of Elements12/1 -> Signal/1
  time/1 -> Natural Frequency Vector/1

== system simulink_model/Nonlinear Dynamic Model/nonlinearity ==
  x : Inport
  Gain3 : Gain  Gain=model.alpha
  Product : Product  Inputs=3
  alpha x ^3 : Outport
  wires:
  Product/1 -> Gain3/1
  Gain3/1 -> alpha x ^3/1
  x/1 -> Product/1, Product/3, Product/2

== system simulink_model/Inner Control Loop/Amplitude Estimator/Buffered Delay2 ==
  note: This block will take an input vector (signal) and output
      | the delayed signal according to a vector delay
  n : Inport
  Constant4 : Constant  Value=round(input.Tn./control.Ts)'
  MATLAB Function1 : MATLAB Function  TreatAsAtomicUnit=on
  n-k : Outport
  wires:
  Constant4/1 -> MATLAB Function1/2(delay_vec)
  n/1 -> MATLAB Function1/1(signal)
  MATLAB Function1/1(y) -> n-k/1  "A_n-k"

== system simulink_model/Inner Control Loop/Nonlinear Dynamic Model1/nonlinearity ==
  x : Inport
  Gain3 : Gain  Gain=model.alpha
  Product : Product  Inputs=3
  alpha x ^3 : Outport
  wires:
  Product/1 -> Gain3/1
  Gain3/1 -> alpha x ^3/1
  x/1 -> Product/1, Product/3, Product/2

== matlab function simulink_model/Amplitude Estimator/Buffered Delay2/MATLAB Function1 ==
  settings: updateMethod=DISCRETE  sampleTime=control.Ts
  data: signal input; y output; delay_vec input
function y = vector_discrete_delay(signal, delay_vec)
% Implements an element-wise discrete delay for a vector signal.
%
% Inputs:
%   signal     - Input signal vector (size N)
%   delay_vec  - Vector specifying delay in discrete sample steps for each element
%
% Output:
%   y          - Delayed output vector (same size as signal)

    % Determine the maximum required delay steps
    maxDelay = max(delay_vec);

    % Ensure persistent buffer for storing past values
    persistent buffer;
    persistent initialized;

    if isempty(initialized)
        % Initialize buffer (rows: time steps, cols: signal elements)
        buffer = zeros(maxDelay + 1, length(signal));
        initialized = true;
    end
    
    y = zeros(size(signal));  % Initialize output
    
    % Shift buffer (push new values to the top, discard oldest)
    buffer = [signal'; buffer(1:end-1, :)];

    % Ensure delay values are within limits
    delay_vec = min(max(delay_vec, 0), maxDelay);

    % Get delayed values
    for i = 1:length(signal)
        y(i) = buffer(delay_vec(i) + 1, i);
    end

end

== matlab function simulink_model/Amplitude Estimator1/Buffered Delay2/MATLAB Function1 ==
  settings: updateMethod=DISCRETE  sampleTime=control.Ts
  data: signal input; y output; delay_vec input
function y = vector_discrete_delay(signal, delay_vec)
% Implements an element-wise discrete delay for a vector signal.
%
% Inputs:
%   signal     - Input signal vector (size N)
%   delay_vec  - Vector specifying delay in discrete sample steps for each element
%
% Output:
%   y          - Delayed output vector (same size as signal)

    % Determine the maximum required delay steps
    maxDelay = max(delay_vec);

    % Ensure persistent buffer for storing past values
    persistent buffer;
    persistent initialized;

    if isempty(initialized)
        % Initialize buffer (rows: time steps, cols: signal elements)
        buffer = zeros(maxDelay + 1, length(signal));
        initialized = true;
    end
    
    y = zeros(size(signal));  % Initialize output
    
    % Shift buffer (push new values to the top, discard oldest)
    buffer = [signal'; buffer(1:end-1, :)];

    % Ensure delay values are within limits
    delay_vec = min(max(delay_vec, 0), maxDelay);

    % Get delayed values
    for i = 1:length(signal)
        y(i) = buffer(delay_vec(i) + 1, i);
    end

end

== matlab function simulink_model/Inner Control Loop/Amplitude Estimator/Buffered Delay2/MATLAB Function1 ==
  settings: updateMethod=DISCRETE  sampleTime=control.Ts
  data: signal input; y output; delay_vec input
function y = vector_discrete_delay(signal, delay_vec)
% Implements an element-wise discrete delay for a vector signal.
%
% Inputs:
%   signal     - Input signal vector (size N)
%   delay_vec  - Vector specifying delay in discrete sample steps for each element
%
% Output:
%   y          - Delayed output vector (same size as signal)

    % Determine the maximum required delay steps
    maxDelay = max(delay_vec);

    % Ensure persistent buffer for storing past values
    persistent buffer;
    persistent initialized;

    if isempty(initialized)
        % Initialize buffer (rows: time steps, cols: signal elements)
        buffer = zeros(maxDelay + 1, length(signal));
        initialized = true;
    end
    
    y = zeros(size(signal));  % Initialize output
    
    % Shift buffer (push new values to the top, discard oldest)
    buffer = [signal'; buffer(1:end-1, :)];

    % Ensure delay values are within limits
    delay_vec = min(max(delay_vec, 0), maxDelay);

    % Get delayed values
    for i = 1:length(signal)
        y(i) = buffer(delay_vec(i) + 1, i);
    end

end
